simulink model "ICs_non_Zero_2ODE_EX3"  (Simulink 8.0)
settings: Solver=ode45  StartTime=1  StopTime=50.0  RelTol=1e-5
PreLoadFcn:
  | K=4;
InitFcn:
  | K=4;
settings Model: Creator=David  LastModifiedBy=David
settings DataIOCC: SignalLoggingSaveFormat=ModelDataLogs
settings DebuggingCC: FcnCallInpInsideContextMsg=UseLocalSettings
settings GRTTargetCC: CombineOutputUpdateFcns=off  GRTInterface=on

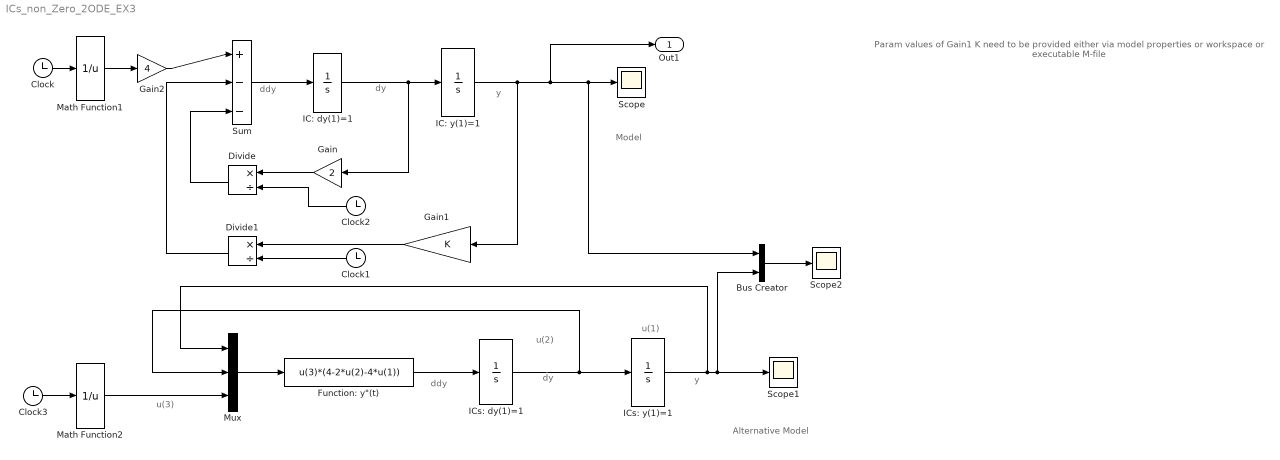
== system ICs_non_Zero_2ODE_EX3 ==
  note: ddy
  note: dy
  note: y
  note: u(3)
  note: u(2)
  note: u(1)
  note: ddy
  note: dy
  note: y
  note: Model
  note: Alternative Model
  note: Param values of Gain1 K need to be provided either via
      | model properties or
      | workspace or
      | executable M-file
  Bus Creator : BusCreator  Inputs=2
  Clock{,1..3} (4 alike) : Clock
  Divide : Product  Inputs=*/
  Divide1 : Product  Inputs=*/
  "Function: y\"(t)" : Fcn  Expr=u(3)*(4-2*u(2)-4*u(1))
  Gain : Gain  Gain=2
  Gain1 : Gain  Gain=K
  Gain2 : Gain  Gain=4
  IC: dy(1)=1 : Integrator  InitialCondition=1
  IC: y(1)=1 : Integrator  InitialCondition=1  UpperSaturationLimit=1  LowerSaturationLimit=0
  ICs: dy(1)=1 : Integrator  InitialCondition=1
  ICs: y(1)=1 : Integrator  InitialCondition=1  UpperSaturationLimit=1  LowerSaturationLimit=0
  Math Function1 : Math  Operator=reciprocal  SaturateOnIntegerOverflow=on
  Math Function2 : Math  Operator=reciprocal  SaturateOnIntegerOverflow=on
  Mux : Mux  Inputs=3
  Scope : Scope
      settings: SaveName=SIM_outs  MaxDataPoints=500000
  Scope1 : Scope
      settings: SaveName=SIM_outs1  MaxDataPoints=500000
  Scope2 : Scope
      settings: SaveName=SIM_outs2  MaxDataPoints=500000
  Sum : Sum  Inputs=|+|--
  Out1 : Outport
  wires:
  IC: dy(1)=1/1 -> IC: y(1)=1/1, Gain/1
  Sum/1 -> IC: dy(1)=1/1
  IC: y(1)=1/1 -> Scope/1, Bus Creator/1, Out1/1, Gain1/1
  Gain2/1 -> Sum/1
  Clock/1 -> Math Function1/1
  Math Function1/1 -> Gain2/1
  Gain/1 -> Divide/1
  Gain1/1 -> Divide1/1
  Clock1/1 -> Divide1/2
  Clock2/1 -> Divide/2
  Divide/1 -> Sum/3
  Divide1/1 -> Sum/2
  Clock3/1 -> Math Function2/1
  Math Function2/1 -> Mux/3
  Mux/1 -> "Function: y\"(t)"/1
  "Function: y\"(t)"/1 -> ICs: dy(1)=1/1
  ICs: dy(1)=1/1 -> ICs: y(1)=1/1, Mux/2
  ICs: y(1)=1/1 -> Mux/1, Scope1/1, Bus Creator/2
  Bus Creator/1 -> Scope2/1
